simulink model "untitled"  (R2016a)
settings: Solver=FixedStepAuto  StartTime=0.0  StopTime=inf  FixedStep=0.001  RelTol=1e-3
libraries: arduinolib x9
settings Model: SimulationMode=external  ExtModeTrigDuration=2  Creator=User  LastModifiedBy=User
settings OptimizationCC: OptimizeModelRefInitCode=on  LifeSpan=1  MaxStackSize=64
settings HardwareCC: ProdBitPerInt=16  ProdBitPerPointer=16  ProdLargestAtomicFloat=None  ProdWordSize=8  ProdHWDeviceType=Atmel->AVR
settings RTWCC: SystemTargetFile=ert.tlc  HardwareBoard=Arduino Uno  TemplateMakefile=ert_default_tmf  Toolchain=Arduino AVR v1.6.1  BuildConfiguration=Faster Runs
settings CodeAppCC: ForceParamTrailComments=on  IgnoreCustomStorageClasses=off  OperatorAnnotations=on  SimulinkDataObjDesc=on  SFDataObjDesc=on  MATLABFcnDesc=on  MangleLength=10  InsertBlockDesc=on  MATLABSourceComments=on
settings ERTTargetCC: SupportContinuousTime=on  SupportVariableSizeSignals=on  ExtMode=on  ExtModeTransport=3  ExtModeMexFile=ext_serial_win32_comm_rtt  ExtModeMexArgs=0 5 115200

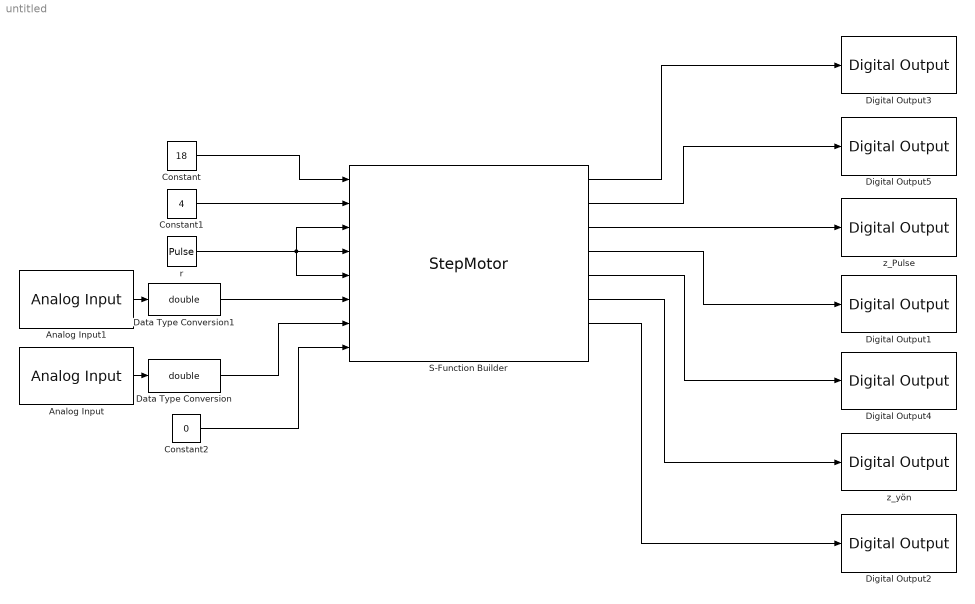
== system untitled ==
  Analog Input : arduinolib/Analog Input  pinNumber=2  sampleTime=0.001  blockPlatform=arduino
  Analog Input1 : arduinolib/Analog Input  pinNumber=1  sampleTime=0.001  blockPlatform=arduino
  Constant : Constant  Value=18
  Constant1 : Constant  Value=4
  Constant2 : Constant  Value=0
  Data Type Conversion : DataTypeConversion  OutDataTypeStr=double
  Data Type Conversion1 : DataTypeConversion  OutDataTypeStr=double
  Digital Output1 : arduinolib/Digital Output  pinNumber=5  blockPlatform=arduino
  Digital Output2 : arduinolib/Digital Output  pinNumber=8  blockPlatform=arduino
  Digital Output3 : arduinolib/Digital Output  pinNumber=2  blockPlatform=arduino
  Digital Output4 : arduinolib/Digital Output  pinNumber=6  blockPlatform=arduino
  Digital Output5 : arduinolib/Digital Output  pinNumber=3  blockPlatform=arduino
  S-Function Builder : S-Function  InitFcn=try, set_param(gcb,'FunctionName','StepMotor'), end  FunctionName=StepMotor  SFunctionModules=StepMotor_wrapper  SFunctionDeploymentMode=off  EnableBusSupport=off  mask(S-Function Builder){}
      mask help: Simulink:masks:SFunctionBuilder_MD
      mask init:
      | val = [[.9  0.75 0.75 1 1 .9 .9 1]',[1 1 0.75 0.75 .9 .9 1 .9]'];try , sys = get_param(gcb,'SfunBuilderFcnName');if isempty(sys), sys = get_param(gcb,'FunctionName'); end,catch, sys = get_param(gcb,'FunctionName'); end
      settings: CopyFcn=set_param(gcbh,'LinkStatus','none')  PreSaveFcn=try, set_param(gcb,'FunctionName','StepMotor'), end  OpenFcn=sfunctionwizard(gcbh)
      mask Display: plot(val(:,1),val(:,2)),disp(sys), port_label('input',1,'x_target'), port_label('input',2,'y_target'), port_label('input',3,'x_pulse'), port_label('input',4,'y_pulse'), port_label('input',5,'z_pulse'), port_label('input',6,'x_limit'), port_label('input',7,'y_limit'), port_label('input',8,'z_input'), port_label('output',1,'x_step'), port_label('output',2,'y_step'), port_label('output',3,'z_step'), port_label('output',4,'x_dir'), port_label('output',5,'y_dir'), port_label('output',6,'z_dir'), port_label('output',7,'enable'), port_label('output',8,'index')
  r : DiscretePulseGenerator  Amplitude=5  SampleTime=0.001
  "z_Pulse " : arduinolib/Digital Output  pinNumber=4  blockPlatform=arduino
  "z_yön " : arduinolib/Digital Output  pinNumber=7  blockPlatform=arduino
  wires:
  Constant/1 -> S-Function Builder/1
  r/1 -> S-Function Builder/5, S-Function Builder/4, S-Function Builder/3
  Constant1/1 -> S-Function Builder/2
  Analog Input1/1 -> Data Type Conversion1/1
  Analog Input/1 -> Data Type Conversion/1
  Data Type Conversion/1 -> S-Function Builder/7
  Data Type Conversion1/1 -> S-Function Builder/6
  S-Function Builder/3 -> "z_Pulse "/1
  S-Function Builder/4 -> Digital Output1/1
  S-Function Builder/2 -> Digital Output5/1
  S-Function Builder/1 -> Digital Output3/1
  S-Function Builder/5 -> Digital Output4/1
  S-Function Builder/6 -> "z_yön "/1
  S-Function Builder/7 -> Digital Output2/1
  Constant2/1 -> S-Function Builder/8
